simulink model "sim12ex3"  (Simulink 4.00)
settings: Solver=ode45  SolverMode=SingleTasking  StartTime=0.0  StopTime=10  MaxStep=.1  RelTol=1e-3  AbsTol=1e-3
settings Model: LastModifiedBy=saadat  SaveTime=off  SaveOutput=off  LimitDataPoints=off  RTWTemplateMakefile=grt_vc.tmf  ExtModeTrigMode=oneshot  ExtModeArmWhenConnect=off

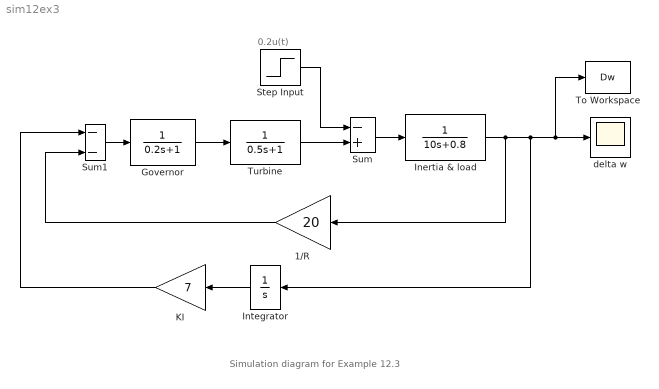
== system sim12ex3 ==
  note: 0.2u(t)
  note: Simulation diagram for Example 12.3
  1/R : Gain  Orientation=left  Gain=20  Multiplication=Element-wise(K.*u)  SaturateOnIntegerOverflow=on
  Governor : TransferFcn  Numerator=[1]  Denominator="[0.2   1]"  AbsoluteTolerance=auto  Realization=auto
  Inertia & load : TransferFcn  Numerator=[1]  Denominator="[10  0.8]"  AbsoluteTolerance=auto  Realization=auto
  Integrator : Integrator  Orientation=left  ExternalReset=none  InitialConditionSource=internal  InitialCondition=0  LimitOutput=off  UpperSaturationLimit=inf  LowerSaturationLimit=-inf  ShowSaturationPort=off  ShowStatePort=off  AbsoluteTolerance=auto
  KI : Gain  Orientation=left  Gain=7  Multiplication=Element-wise(K.*u)  SaturateOnIntegerOverflow=on
  Step Input : Step  Time=0  Before=0  After=.2  SampleTime=0
  Sum : Sum  Inputs=-+  SaturateOnIntegerOverflow=on
  Sum1 : Sum  Inputs=--  SaturateOnIntegerOverflow=on
  To Workspace : ToWorkspace  VariableName=Dw  SampleTime=0  SaveFormat=Array
      settings: MaxDataPoints=1000
  Turbine : TransferFcn  Numerator=[1]  Denominator="[0.5  1]"  AbsoluteTolerance=auto  Realization=auto
  delta w : Scope
      settings: TickLabels=on  TimeRange=10  YMin=-0.015  YMax=0.005  SaveToWorkspace=off  SaveName=ScopeData  DataFormat=Array  LimitDataPoints=on  MaxDataPoints=5000
  wires:
  Governor/1 -> Turbine/1
  Turbine/1 -> Sum/2
  Sum/1 -> Inertia & load/1
  Sum1/1 -> Governor/1
  Integrator/1 -> KI/1
  KI/1 -> Sum1/1
  1/R/1 -> Sum1/2
  Step Input/1 -> Sum/1
  Inertia & load/1 -> 1/R/1, Integrator/1, delta w/1, To Workspace/1
